simulink model "clockRatePipelining"  (R2024a)
settings: Solver=FixedStepDiscrete  StartTime=0.0  StopTime=100/100e6  RelTol=1e-3
settings Model: DataTypeOverride=Off  Creator=cotti  LastModifiedBy=cotti
settings OptimizationCC: BlockReduction=off  ConditionallyExecuteInputs=off  DefaultParameterBehavior=Inlined  InheritOutputTypeSmallerThanSingle=on
settings DebuggingCC: AlgebraicLoopMsg=error  ArtificialAlgebraicLoopMsg=error  SingleTaskRateTransMsg=error  UnconnectedInputMsg=warning  UnconnectedOutputMsg=warning  UnconnectedLineMsg=warning
settings HardwareCC: ProdBitPerPointer=32  ProdBitPerSizeT=32  ProdBitPerPtrDiffT=32  ProdLargestAtomicFloat=None  ProdIntDivRoundTo=Undefined  ProdEndianess=Unspecified  ProdWordSize=32  ProdHWDeviceType=ASIC/FPGA->ASIC/FPGA  TargetBitPerLong=64  TargetBitPerPointer=64  TargetBitPerSizeT=64  TargetBitPerPtrDiffT=64  TargetLongLongMode=on  TargetIntDivRoundTo=Zero  TargetEndianess=LittleEndian  TargetWordSize=64  TargetHWDeviceType=Custom Processor->MATLAB Host Computer  ProdEqTarget=off

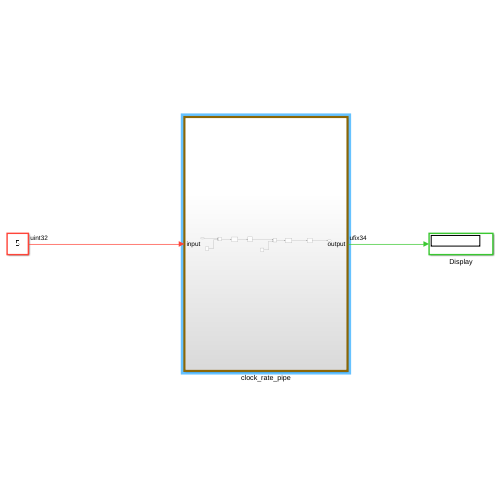
[thumbnail: Simulink's stored preview of the top-level diagram]
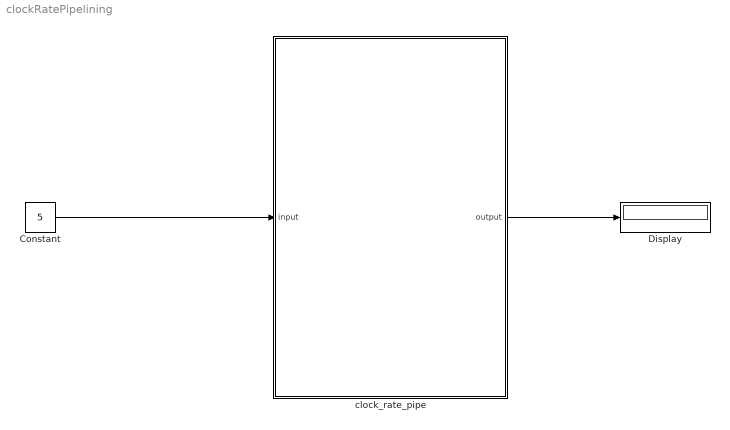
== system clockRatePipelining ==
  Constant : Constant  Value=5  OutDataTypeStr=uint32  SampleTime=1/100e6
  Display : Display
  clock_rate_pipe : Subsystem  TreatAsAtomicUnit=on
  wires:
  Constant/1 -> clock_rate_pipe/1(input)
  clock_rate_pipe/1(output) -> Display/1

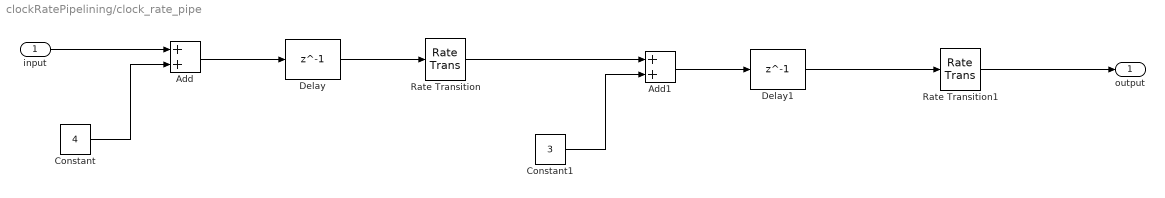
== system clockRatePipelining/clock_rate_pipe ==
  input : Inport
  Add : Sum
  Add1 : Sum
  Constant : Constant  Value=4  OutDataTypeStr=uint32  SampleTime=1/100e6
  Constant1 : Constant  Value=3  OutDataTypeStr=uint32  SampleTime=1/50e6
  Delay : Delay  DelayLength=1  InitialCondition=0  UseCircularBuffer=on
  Delay1 : Delay  DelayLength=1  InitialCondition=0  UseCircularBuffer=on
  Rate Transition : RateTransition  OutPortSampleTime=1/50e6
  Rate Transition1 : RateTransition  OutPortSampleTime=1/100e6
  output : Outport
  wires:
  Delay/1 -> Rate Transition/1
  Add/1 -> Delay/1
  input/1 -> Add/1
  Constant/1 -> Add/2
  Constant1/1 -> Add1/2
  Rate Transition/1 -> Add1/1
  Add1/1 -> Delay1/1
  Delay1/1 -> Rate Transition1/1
  Rate Transition1/1 -> output/1
